simulink model "Lab1"  (R2021a)
settings: Solver=VariableStepAuto  StartTime=0.0  StopTime=30  RelTol=1e-3
values from neighbouring files (symbols this model uses):
  A = zeros(2,2)    [initializare_model.m]
  B = zeros(2,4)    [initializare_model.m]
  C = eye(2)    [initializare_model.m]
  c0 = 5.4698    [initializare_model.m]
  ci = 10    [initializare_model.m]
  D = zeros(2,4)    [initializare_model.m]
  EdR = 49584/8.32    (= 5959.61538462)    [initializare_model.m]
  hA = kT*At    (= 18821.555234)    [initializare_model.m]
  k0 = 34930800    [initializare_model.m]
  mdH = 24953    [initializare_model.m]
  q = 10    [initializare_model.m]
  rcp = 2093    [initializare_model.m]
  T0 = 339.437    [initializare_model.m]
  Ti = 38+273    (= 311)    [initializare_model.m]
  Tri = 38+273    (= 311)    [initializare_model.m]
  V = 10    [initializare_model.m]
settings Model: Creator=Automatica  LastModifiedBy=Automatica

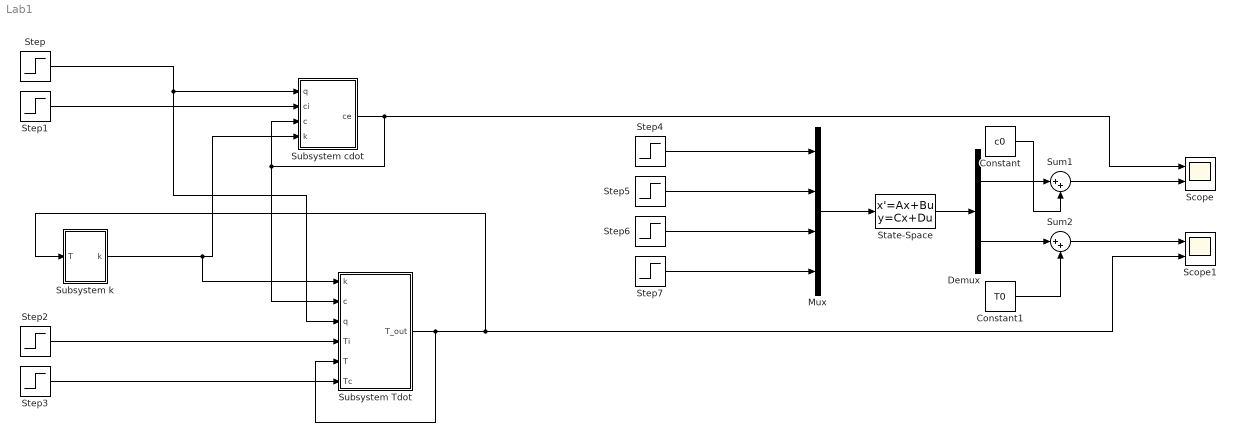
== system Lab1 ==
  Constant : Constant  Value=c0
  Constant1 : Constant  Value=T0
  Demux : Demux  Outputs=2
  Mux : Mux
  Scope : Scope  NumInputPorts=2
  Scope1 : Scope  NumInputPorts=2
  State-Space : StateSpace  A=A  B=B  C=C  D=D  InitialCondition=0
  Step : Step  Time=0  Before=1.5*q  After=1.5*q  SampleTime=0
  Step1 : Step  Time=0  Before=ci  After=ci  SampleTime=0
  Step2 : Step  Time=0  Before=Ti  After=Ti  SampleTime=0
  Step3 : Step  Time=0  Before=Tri  After=Tri  SampleTime=0
  Step4 : Step  Time=0  Before=0.5*q  After=0.5*q  SampleTime=0
  Step5 : Step  Time=0  After=0  SampleTime=0
  Step6 : Step  Time=0  After=0  SampleTime=0
  Step7 : Step  Time=0  After=0  SampleTime=0
  Subsystem Tdot : Subsystem
  Subsystem cdot : Subsystem
  Subsystem k : Subsystem
  Sum1 : Sum  Inputs=|++
  Sum2 : Sum  Inputs=|++
  wires:
  Step/1 -> Subsystem Tdot/3(q), Subsystem cdot/1(q)
  Step1/1 -> Subsystem cdot/2(ci)
  Subsystem k/1(k) -> Subsystem Tdot/1(k), Subsystem cdot/4(k)
  Subsystem cdot/1(ce) -> Scope/1, Subsystem cdot/3(c), Subsystem Tdot/2(c)
  Subsystem Tdot/1(T_out) -> Subsystem Tdot/5(T), Scope1/2, Subsystem k/1(T)
  Step3/1 -> Subsystem Tdot/6(Tc)
  Step2/1 -> Subsystem Tdot/4(Ti)
  Step4/1 -> Mux/1
  Step5/1 -> Mux/2
  Step6/1 -> Mux/3
  Step7/1 -> Mux/4
  Mux/1 -> State-Space/1
  State-Space/1 -> Demux/1
  Demux/1 -> Sum1/1
  Constant/1 -> Sum1/2
  Demux/2 -> Sum2/1
  Constant1/1 -> Sum2/2
  Sum1/1 -> Scope/2
  Sum2/1 -> Scope1/1

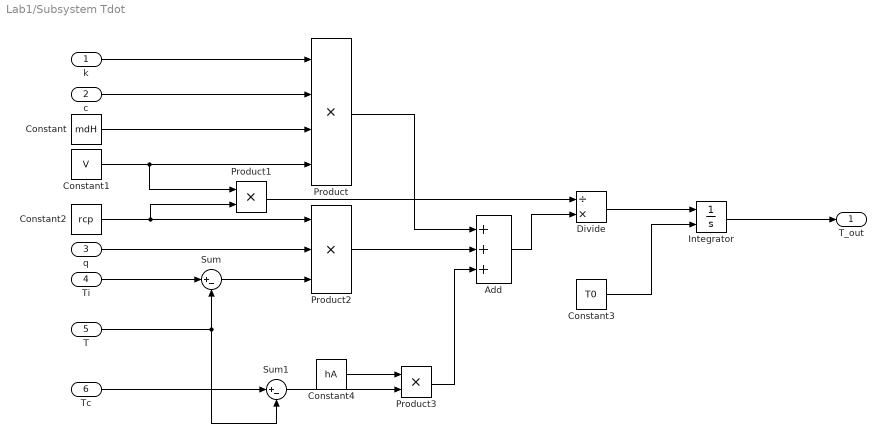
== system Lab1/Subsystem Tdot ==
  k : Inport
  c : Inport  Port=2
  q : Inport  Port=3
  Ti : Inport  Port=4
  T : Inport  Port=5
  Tc : Inport  Port=6
  Add : Sum  Inputs=+++
  Constant : Constant  Value=mdH
  Constant1 : Constant  Value=V
  Constant2 : Constant  Value=rcp
  Constant3 : Constant  Value=T0
  Constant4 : Constant  Value=hA
  Divide : Product  Inputs=/*
  Integrator : Integrator  InitialConditionSource=external
  Product : Product  Inputs=4
  Product1 : Product
  Product2 : Product  Inputs=3
  Product3 : Product
  Sum : Sum  Inputs=|+-
  Sum1 : Sum  Inputs=|+-
  T_out : Outport
  wires:
  Tc/1 -> Sum1/1
  T/1 -> Sum1/2, Sum/2
  Ti/1 -> Sum/1
  k/1 -> Product/1
  c/1 -> Product/2
  Constant/1 -> Product/3
  Constant1/1 -> Product1/1, Product/4
  Constant2/1 -> Product2/1, Product1/2
  q/1 -> Product2/2
  Sum/1 -> Product2/3
  Product1/1 -> Divide/1
  Product2/1 -> Add/2
  Product/1 -> Add/1
  Add/1 -> Divide/2
  Divide/1 -> Integrator/1
  Sum1/1 -> Product3/2
  Constant4/1 -> Product3/1
  Product3/1 -> Add/3
  Constant3/1 -> Integrator/2
  Integrator/1 -> T_out/1

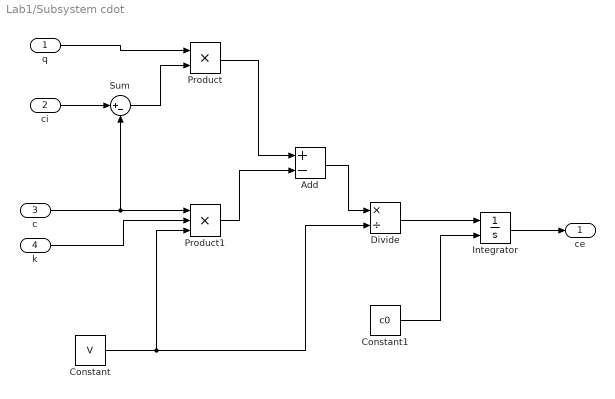
== system Lab1/Subsystem cdot ==
  q : Inport
  ci : Inport  Port=2
  c : Inport  Port=3
  k : Inport  Port=4
  Add : Sum  Inputs=+-
  Constant : Constant  Value=V
  Constant1 : Constant  Value=c0
  Divide : Product  Inputs=*/
  Integrator : Integrator  InitialConditionSource=external
  Product : Product
  Product1 : Product  Inputs=3
  Sum : Sum  Inputs=|+-
  ce : Outport
  wires:
  ci/1 -> Sum/1
  Sum/1 -> Product/2
  q/1 -> Product/1
  Product/1 -> Add/1
  Product1/1 -> Add/2
  c/1 -> Sum/2, Product1/1
  k/1 -> Product1/2
  Constant/1 -> Product1/3, Divide/2
  Add/1 -> Divide/1
  Divide/1 -> Integrator/1
  Constant1/1 -> Integrator/2
  Integrator/1 -> ce/1

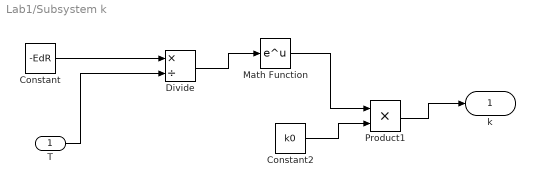
== system Lab1/Subsystem k ==
  T : Inport
  Constant : Constant  Value=-EdR
  Constant2 : Constant  Value=k0
  Divide : Product  Inputs=*/
  Math Function : Math  SaturateOnIntegerOverflow=on
  Product1 : Product
  k : Outport
  wires:
  Constant/1 -> Divide/1
  T/1 -> Divide/2
  Constant2/1 -> Product1/2
  Product1/1 -> k/1
  Math Function/1 -> Product1/1
  Divide/1 -> Math Function/1
